simulink model "baseline_super"  (R2021a)
settings: Solver=FixedStepAuto  StartTime=0.0  StopTime=50  FixedStep=framePeriod_s  RelTol=1e-3
undefined symbols (not defined in the file or in its folder): Aircraft, Earth, framePeriod_s, WGS84
libraries: pid_lib x32, simulink x29, aerolibtransform2 x3, simulink_extras x2, aerolibguid x1
(part 2 of 4)

== system baseline_super/RTL CONTROLLER/Horizontal_position_controller ==
  dist_to_tar_m : Inport
  bearing_to_tar_rad : Inport  Port=2
  cur_heading_rad : Inport  Port=3
  Constant : Constant  Value=0  OutDataTypeStr=single
  Constant1 : Constant  Value=Aircraft.Control.v_hor_max  OutDataTypeStr=single
  Constant3 : Constant  Value=0.5  OutDataTypeStr=single
  Mux : Mux  Inputs=2
  PID Controller2 : pid_lib/PID Controller  Controller=P  Form=Parallel  TimeDomain=Discrete-time  UseExternalTs=off  SampleTime=framePeriod_s  IntegratorMethod=Forward Euler  FilterMethod=Forward Euler  ControllerParametersSource=external  P=0.335  I=0.005  D=0  UseFilter=off  N=100  TunerSelectOption=Transfer Function Based (PID Tuner App)  InitialConditionSource=internal  InitialConditionForIntegrator=0  InitialConditionForFilter=0  DifferentiatorICPrevScaledInput=0  ExternalReset=none  TrackingMode=off  Kt=1  LimitOutput=on  SatLimitsSource=external  UpperSaturationLimit=inf  LowerSaturationLimit=-inf  LinearizeAsGain=off  AntiWindupMode=clamping  Kb=1  POutMin=[]  POutMax=[]  IOutMin=[]  IOutMax=[]  DOutMin=[]  DOutMax=[]  NOutMin=[]  NOutMax=[]  SumOutMin=[]  SumOutMax=[]  SaturationOutMin=[]  SaturationOutMax=[]  PParamMin=[]  PParamMax=[]  IParamMin=[]  IParamMax=[]  DParamMin=[]  DParamMax=[]  NParamMin=[]  NParamMax=[]  KbParamMin=[]  KbParamMax=[]  KtParamMin=[]  KtParamMax=[]  KbOutMin=[]  KbOutMax=[]  KtOutMin=[]  KtOutMax=[]  IntegratorOutMin=[]  IntegratorOutMax=[]  FilterOutMin=[]  FilterOutMax=[]  SumI1OutMin=[]  SumI1OutMax=[]  SumI2OutMin=[]  SumI2OutMax=[]  SumI3OutMin=[]  SumI3OutMax=[]  SumI4OutMin=[]  SumI4OutMax=[]  SumDOutMin=[]  SumDOutMax=[]  DifferentiatorOutMin=[]  DifferentiatorOutMax=[]  FilterDiffOutCoefMin=[]  FilterDiffOutCoefMax=[]  ReciprocalOutMin=[]  ReciprocalOutMax=[]  SumDenOutMin=[]  SumDenOutMax=[]  SumNumOutMin=[]  SumNumOutMax=[]  DivideOutMin=[]  DivideOutMax=[]  UdiffTsProdOutMin=[]  UdiffTsProdOutMax=[]  NTsProdOutMin=[]  NTsProdOutMax=[]  UintegralTsProdOutMin=[]  UintegralTsProdOutMax=[]  UngainTsProdOutMin=[]  UngainTsProdOutMax=[]  IntegratorContinuousStateAttributes=''  IntegratorStateMustResolveToSignalObject=off  IntegratorRTWStateStorageClass=Auto  FilterContinuousStateAttributes=''  FilterStateMustResolveToSignalObject=off  FilterRTWStateStorageClass=Auto  ParallelPVariant=ExternalParameters  IdealPVariant=Disabled  IVariant=Disabled  DVariant=Disabled  IntegratorVariant=Disabled  SatVariant=External  AWVariant=Disabled  PCopyVariant=Disabled  TRVariant=Disabled  FdbkBlocksVariant=Forward  IdealPFdbkVariant=Disabled  SatFdbkVariant=Disabled  DerivativeFilterVariant=Disabled  NVariant=Disabled  NCopyVariant=Disabled_SignalSpec  FilterICVariant=Disabled  IntegratorICVariant=Disabled  ExternalResetVariant=Disabled  TRSumVariant=Passthrough  SumFdbkVariant=Disabled  SumVariant=Passthrough_P  TsampFilterVariant=InternalTs  TsampNgainVariant=Passthrough  TsampIntegralVariant=Disabled_SignalSpec  ExternalSaturationOutDataTypeStr=Inherit: Same as second input
  Saturation : Saturate  UpperLimit=20  LowerLimit=0
  convert to ve_cmd : Subsystem
  inertial_to_body conversion : Subsystem
  vb_x : Outport
  vb_y : Outport  Port=2
  wires:
  Constant3/1 -> PID Controller2/2
  cur_heading_rad/1 -> inertial_to_body conversion/2(heading_rad)
  bearing_to_tar_rad/1 -> convert to ve_cmd/2(bearing_to_target_rad)
  convert to ve_cmd/1(ve_x_cmd) -> Mux/1  "ve_x"
  convert to ve_cmd/2(ve_y_cmd) -> Mux/2  "ve_y"
  Mux/1 -> inertial_to_body conversion/1(ve_xy)
  Constant1/1 -> PID Controller2/3
  Constant/1 -> PID Controller2/4
  PID Controller2/1 -> convert to ve_cmd/1(speed_cmd_mps)
  Saturation/1 -> PID Controller2/1
  dist_to_tar_m/1 -> Saturation/1
  inertial_to_body conversion/1(vb_x) -> vb_x/1
  inertial_to_body conversion/2(vb_y) -> vb_y/1

== system baseline_super/RTL CONTROLLER/Trigger Land ==
  Trigger : TriggerPort  VariantControl=(inherit)  PortDimensions=1
  Data Store Write : DataStoreWrite  DataStoreName=cur_mode  IndexOptions=Index vector (dialog)  Indices=1  OutputSizes=1
  Land_mode : Constant  Value=4  OutDataTypeStr=int8
  wires:
  Land_mode/1 -> Data Store Write/1

== system baseline_super/RTL CONTROLLER/heading_controller ==
  Sys_input : Inport
  Bus Selector4 : BusSelector  OutputSignals=Navigation Filter Data.gyro_radps
  Constant : Constant  Value=0  OutDataTypeStr=single
  Selector2 : Selector  InputPortWidth=3  IndexOptions=Index vector (dialog)  Indices=3  OutputSizes=1
  yaw_rate_controller : Subsystem
  yaw_cc : Outport
  wires:
  Bus Selector4/1 -> Selector2/1  "<gyro_radps>"
  Sys_input/1 -> Bus Selector4/1
  Constant/1 -> yaw_rate_controller/1(yaw_rate_cmd_radps)
  yaw_rate_controller/1(yaw_cmd) -> yaw_cc/1
  Selector2/1 -> yaw_rate_controller/2(gyro_z_radps)

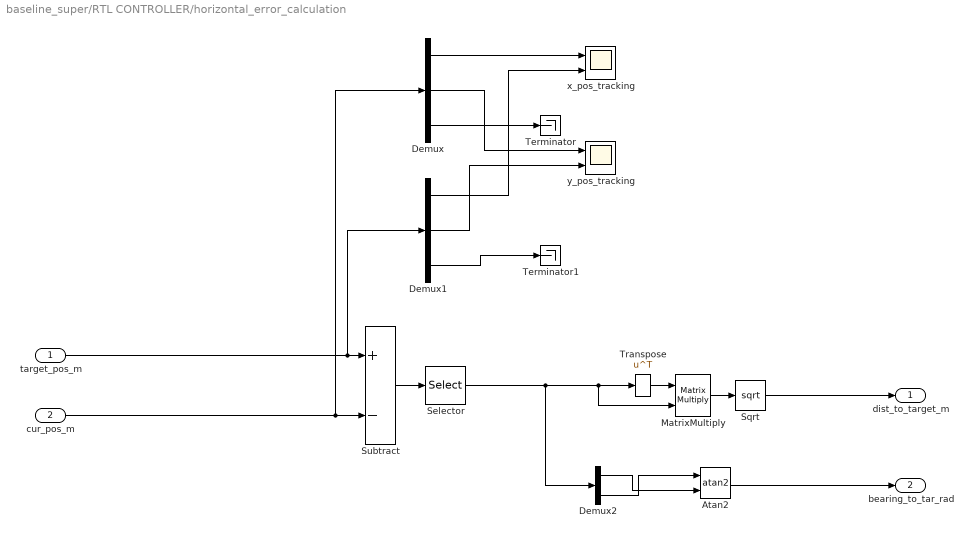
== system baseline_super/RTL CONTROLLER/horizontal_error_calculation  ==
  target_pos_m : Inport
  cur_pos_m : Inport  Port=2
  Atan2 : Trigonometry  Operator=atan2
  Demux : Demux  Outputs=3
  Demux1 : Demux  Outputs=3
  Demux2 : Demux  Outputs=2
  MatrixMultiply : Product  Multiplication=Matrix(*)
  Selector : Selector  InputPortWidth=3  IndexOptions=Index vector (dialog)  Indices=[1 2]  OutputSizes=1
  Sqrt : Sqrt  SaturateOnIntegerOverflow=on
  Subtract : Sum  Inputs=+-
  Terminator : Terminator
  Terminator1 : Terminator
  Transpose : Math  Operator=transpose  SaturateOnIntegerOverflow=on
  x_pos_tracking : Scope  NumInputPorts=2
  y_pos_tracking : Scope  NumInputPorts=2
  dist_to_target_m : Outport
  bearing_to_tar_rad : Outport  Port=2
  wires:
  Demux/3 -> Terminator/1
  Demux/2 -> y_pos_tracking/1
  target_pos_m/1 -> Demux1/1, Subtract/1
  cur_pos_m/1 -> Demux/1, Subtract/2
  Selector/1 -> Demux2/1, MatrixMultiply/2, Transpose/1
  Demux1/3 -> Terminator1/1
  Atan2/1 -> bearing_to_tar_rad/1
  Subtract/1 -> Selector/1
  Demux/1 -> x_pos_tracking/1
  Demux2/2 -> Atan2/1
  Transpose/1 -> MatrixMultiply/1
  Demux1/1 -> x_pos_tracking/2
  Demux1/2 -> y_pos_tracking/2
  MatrixMultiply/1 -> Sqrt/1
  Demux2/1 -> Atan2/2
  Sqrt/1 -> dist_to_target_m/1

== system baseline_super/RTL CONTROLLER/horizontal_speed_controller ==
  vb_x cmd : Inport
  vb_y cmd : Inport  Port=2
  <heading_rad> : Inport  Port=3
  ve_xy : Inport  Port=4
  inertial_to_body conversion : Subsystem
  vb_x_controller : Subsystem
  vb_y_controller : Subsystem
  roll_cmd_rad : Outport
  pitch_cmd_rad : Outport  Port=2
  wires:
  vb_x cmd/1 -> vb_x_controller/1(vb_x cmd)
  vb_y cmd/1 -> vb_y_controller/1(vb_y cmd)
  vb_x_controller/1(pitch_cmd_rad) -> pitch_cmd_rad/1
  vb_y_controller/1(roll_cmd_rad) -> roll_cmd_rad/1
  <heading_rad>/1 -> inertial_to_body conversion/1(<heading_rad>)
  ve_xy/1 -> inertial_to_body conversion/2(ve_xy)
  inertial_to_body conversion/1(vb_y) -> vb_y_controller/2(vb_y)
  inertial_to_body conversion/2(vb_x) -> vb_x_controller/2(vb_x)

== system baseline_super/RTL CONTROLLER/pitch_roll_angle_controller ==
  roll_cmd_rad : Inport
  roll_rad : Inport  Port=2
  pitch_cmd_rad : Inport  Port=3
  pitch_rad : Inport  Port=4
  Pitch Controller : Subsystem
  Roll Controller : Subsystem
  roll_cc : Outport
  pitch_cc : Outport  Port=2
  wires:
  Pitch Controller/1(pitch_cc) -> pitch_cc/1  "pitch_cc"
  pitch_rad/1 -> Pitch Controller/2(pitch_rad)
  Roll Controller/1(roll_cc) -> roll_cc/1  "roll_cc"
  pitch_cmd_rad/1 -> Pitch Controller/1(pitch_cmd_rad)
  roll_cmd_rad/1 -> Roll Controller/1(roll_cmd_rad)
  roll_rad/1 -> Roll Controller/2(roll_rad)

== system baseline_super/RTL CONTROLLER/vertical_position_controller ==
  target_z_m : Inport
  cur_z_m : Inport  Port=2
  Abs : Abs
  Compare To Constant : simulink/Logic and Bit Operations/Compare To Constant  relop=<=  const=Aircraft.Control.wp_radius  OutDataTypeStr=boolean
  Constant : Constant  Value=Aircraft.Control.v_z_up_max  OutDataTypeStr=single
  Constant1 : Constant  Value=Aircraft.Control.v_z_down_max  OutDataTypeStr=single
  Gain : Gain  Gain=-1
  PID Controller2 : pid_lib/PID Controller  Controller=P  Form=Parallel  TimeDomain=Discrete-time  UseExternalTs=off  SampleTime=framePeriod_s  IntegratorMethod=Forward Euler  FilterMethod=Forward Euler  ControllerParametersSource=external  P=0  I=0  D=0  UseFilter=off  N=100  TunerSelectOption=Frequency Response Based  ZeroCross=off  InitialConditionSource=internal  InitialConditionForIntegrator=0  InitialConditionForFilter=0  DifferentiatorICPrevScaledInput=0  ExternalReset=none  TrackingMode=off  Kt=1  LimitOutput=on  SatLimitsSource=external  UpperSaturationLimit=Aircraft.Control.v_z_up_max  LowerSaturationLimit=-Aircraft.Control.v_z_down_max  LinearizeAsGain=on  AntiWindupMode=clamping  Kb=1  POutMin=[]  POutMax=[]  IOutMin=[]  IOutMax=[]  DOutMin=[]  DOutMax=[]  NOutMin=[]  NOutMax=[]  SumOutMin=[]  SumOutMax=[]  SaturationOutMin=[]  SaturationOutMax=[]  PParamMin=[]  PParamMax=[]  IParamMin=[]  IParamMax=[]  DParamMin=[]  DParamMax=[]  NParamMin=[]  NParamMax=[]  KbParamMin=[]  KbParamMax=[]  KtParamMin=[]  KtParamMax=[]  KbOutMin=[]  KbOutMax=[]  KtOutMin=[]  KtOutMax=[]  IntegratorOutMin=[]  IntegratorOutMax=[]  FilterOutMin=[]  FilterOutMax=[]  SumI1OutMin=[]  SumI1OutMax=[]  SumI2OutMin=[]  SumI2OutMax=[]  SumI3OutMin=[]  SumI3OutMax=[]  SumI4OutMin=[]  SumI4OutMax=[]  SumDOutMin=[]  SumDOutMax=[]  DifferentiatorOutMin=[]  DifferentiatorOutMax=[]  FilterDiffOutCoefMin=[]  FilterDiffOutCoefMax=[]  ReciprocalOutMin=[]  ReciprocalOutMax=[]  SumDenOutMin=[]  SumDenOutMax=[]  SumNumOutMin=[]  SumNumOutMax=[]  DivideOutMin=[]  DivideOutMax=[]  UdiffTsProdOutMin=[]  UdiffTsProdOutMax=[]  NTsProdOutMin=[]  NTsProdOutMax=[]  UintegralTsProdOutMin=[]  UintegralTsProdOutMax=[]  UngainTsProdOutMin=[]  UngainTsProdOutMax=[]  IntegratorContinuousStateAttributes=''  IntegratorStateMustResolveToSignalObject=off  IntegratorRTWStateStorageClass=Auto  FilterContinuousStateAttributes=''  FilterStateMustResolveToSignalObject=off  FilterRTWStateStorageClass=Auto  ParallelPVariant=ExternalParameters  IdealPVariant=Disabled  IVariant=Disabled  DVariant=Disabled  IntegratorVariant=Disabled  SatVariant=External  AWVariant=Disabled  PCopyVariant=Disabled  TRVariant=Disabled  FdbkBlocksVariant=Forward  IdealPFdbkVariant=Disabled  SatFdbkVariant=Disabled  DerivativeFilterVariant=Disabled  NVariant=Disabled  NCopyVariant=Disabled_SignalSpec  FilterICVariant=Disabled  IntegratorICVariant=Disabled  ExternalResetVariant=Disabled  TRSumVariant=Passthrough  SumFdbkVariant=Disabled  SumVariant=Passthrough_P  TsampFilterVariant=InternalTs  TsampNgainVariant=Passthrough  TsampIntegralVariant=Disabled_SignalSpec  ExternalSaturationOutDataTypeStr=Inherit: Same as second input
  P_vz1 : Constant  Value=Aircraft.Control.P_alt  OutDataTypeStr=single
  Sum3 : Sum  Inputs=|+-
  ve_z_cmd : Outport
  rtl_alt_cleared : Outport  Port=2
  wires:
  P_vz1/1 -> PID Controller2/2
  target_z_m/1 -> Sum3/1
  Sum3/1 -> Abs/1, PID Controller2/1
  cur_z_m/1 -> Sum3/2
  Constant1/1 -> PID Controller2/3
  Constant/1 -> Gain/1
  Gain/1 -> PID Controller2/4
  PID Controller2/1 -> ve_z_cmd/1
  Compare To Constant/1 -> rtl_alt_cleared/1
  Abs/1 -> Compare To Constant/1

== system baseline_super/RTL CONTROLLER/vertical_speed_controller ==
  ve_z_cmd : Inport
  ve_z_mps : Inport  Port=2
  Constant2 : Constant  Value=Aircraft.Control.est_hover_thr  OutDataTypeStr=single
  D_vz : Constant  Value=Aircraft.Control.D_v_z  OutDataTypeStr=single
  Gain : Gain  Gain=-1
  I_vz : Constant  Value=Aircraft.Control.I_v_z  OutDataTypeStr=single
  PID Controller : pid_lib/PID Controller  Controller=PID  Form=Parallel  TimeDomain=Discrete-time  UseExternalTs=off  SampleTime=framePeriod_s  IntegratorMethod=Forward Euler  FilterMethod=Forward Euler  ControllerParametersSource=external  P=0  I=0  D=0  UseFilter=off  N=100  TunerSelectOption=Frequency Response Based  InitialConditionSource=internal  InitialConditionForIntegrator=0  InitialConditionForFilter=0  DifferentiatorICPrevScaledInput=0  ExternalReset=none  TrackingMode=off  Kt=1  LimitOutput=on  SatLimitsSource=internal  UpperSaturationLimit=inf  LowerSaturationLimit=-inf  LinearizeAsGain=on  AntiWindupMode=clamping  Kb=1  POutMin=[]  POutMax=[]  IOutMin=[]  IOutMax=[]  DOutMin=[]  DOutMax=[]  NOutMin=[]  NOutMax=[]  SumOutMin=[]  SumOutMax=[]  SaturationOutMin=[]  SaturationOutMax=[]  PParamMin=[]  PParamMax=[]  IParamMin=[]  IParamMax=[]  DParamMin=[]  DParamMax=[]  NParamMin=[]  NParamMax=[]  KbParamMin=[]  KbParamMax=[]  KtParamMin=[]  KtParamMax=[]  KbOutMin=[]  KbOutMax=[]  KtOutMin=[]  KtOutMax=[]  IntegratorOutMin=[]  IntegratorOutMax=[]  FilterOutMin=[]  FilterOutMax=[]  SumI1OutMin=[]  SumI1OutMax=[]  SumI2OutMin=[]  SumI2OutMax=[]  SumI3OutMin=[]  SumI3OutMax=[]  SumI4OutMin=[]  SumI4OutMax=[]  SumDOutMin=[]  SumDOutMax=[]  DifferentiatorOutMin=[]  DifferentiatorOutMax=[]  FilterDiffOutCoefMin=[]  FilterDiffOutCoefMax=[]  ReciprocalOutMin=[]  ReciprocalOutMax=[]  SumDenOutMin=[]  SumDenOutMax=[]  SumNumOutMin=[]  SumNumOutMax=[]  DivideOutMin=[]  DivideOutMax=[]  UdiffTsProdOutMin=[]  UdiffTsProdOutMax=[]  NTsProdOutMin=[]  NTsProdOutMax=[]  UintegralTsProdOutMin=[]  UintegralTsProdOutMax=[]  UngainTsProdOutMin=[]  UngainTsProdOutMax=[]  IntegratorContinuousStateAttributes=''  IntegratorStateMustResolveToSignalObject=off  IntegratorRTWStateStorageClass=Auto  FilterContinuousStateAttributes=''  FilterStateMustResolveToSignalObject=off  FilterRTWStateStorageClass=Auto  ParallelPVariant=ExternalParameters  IdealPVariant=Disabled  IVariant=ExternalParameters  DVariant=ExternalParameters  IntegratorVariant=Discrete  SatVariant=Enabled  AWVariant=DiscClampingParallel  PCopyVariant=Disabled  TRVariant=Disabled  FdbkBlocksVariant=Forward  IdealPFdbkVariant=Disabled  SatFdbkVariant=Disabled  DerivativeFilterVariant=Differentiator  NVariant=Passthrough  NCopyVariant=Disabled_SignalSpec  FilterICVariant=InternalICsDifferentiator  IntegratorICVariant=InternalICs  ExternalResetVariant=Disabled  TRSumVariant=Passthrough  SumFdbkVariant=Disabled  SumVariant=Sum_PID  TsampFilterVariant=InternalTs  TsampNgainVariant=Passthrough  TsampIntegralVariant=Passthrough  ExternalSaturationOutDataTypeStr=Inherit: Same as second input
  P_vz : Constant  Value=Aircraft.Control.P_v_z  OutDataTypeStr=single
  Saturation : Saturate  UpperLimit=1  LowerLimit=0
  Sum : Sum  Inputs=|+-
  Sum1 : Sum  Inputs=|++
  throttle : Outport
  wires:
  Sum/1 -> Gain/1  "error"
  Constant2/1 -> Sum1/2
  D_vz/1 -> PID Controller/4
  ve_z_mps/1 -> Sum/2
  I_vz/1 -> PID Controller/3
  Sum1/1 -> Saturation/1
  P_vz/1 -> PID Controller/2
  PID Controller/1 -> Sum1/1
  ve_z_cmd/1 -> Sum/1
  Saturation/1 -> throttle/1  "throttle"
  Gain/1 -> PID Controller/1

== system baseline_super/STABILIZED CONTROLER/Pitch Controller ==
  Pitch Bus : Inport
  Pitch_cmd : Inport  Port=2
  Bus Selector : BusSelector  OutputSignals=Navigation Filter Data.pitch_rad
  Constant : Constant  Value=Aircraft.Control.P_pitch_angle  OutDataTypeStr=single
  Constant1 : Constant  Value=Aircraft.Control.I_pitch_angle  OutDataTypeStr=single
  Constant2 : Constant  Value=Aircraft.Control.D_pitch_angle  OutDataTypeStr=single
  Mux : Mux  Inputs=2
  pitch_norm_to_actual : Gain  Gain=-Aircraft.Control.pitch_angle_lim
  stab_pitch_PID : pid_lib/PID Controller  Controller=PID  Form=Parallel  TimeDomain=Discrete-time  UseExternalTs=off  SampleTime=framePeriod_s  IntegratorMethod=Forward Euler  FilterMethod=Forward Euler  ControllerParametersSource=external  P=0.335  I=0.005  D=0  UseFilter=off  N=100  TunerSelectOption=Transfer Function Based (PID Tuner App)  InitialConditionSource=internal  InitialConditionForIntegrator=0  InitialConditionForFilter=0  DifferentiatorICPrevScaledInput=0  ExternalReset=none  TrackingMode=off  Kt=1  LimitOutput=on  SatLimitsSource=internal  UpperSaturationLimit=inf  LowerSaturationLimit=-inf  LinearizeAsGain=on  AntiWindupMode=clamping  Kb=1  POutMin=[]  POutMax=[]  IOutMin=[]  IOutMax=[]  DOutMin=[]  DOutMax=[]  NOutMin=[]  NOutMax=[]  SumOutMin=[]  SumOutMax=[]  SaturationOutMin=[]  SaturationOutMax=[]  PParamMin=[]  PParamMax=[]  IParamMin=[]  IParamMax=[]  DParamMin=[]  DParamMax=[]  NParamMin=[]  NParamMax=[]  KbParamMin=[]  KbParamMax=[]  KtParamMin=[]  KtParamMax=[]  KbOutMin=[]  KbOutMax=[]  KtOutMin=[]  KtOutMax=[]  IntegratorOutMin=[]  IntegratorOutMax=[]  FilterOutMin=[]  FilterOutMax=[]  SumI1OutMin=[]  SumI1OutMax=[]  SumI2OutMin=[]  SumI2OutMax=[]  SumI3OutMin=[]  SumI3OutMax=[]  SumI4OutMin=[]  SumI4OutMax=[]  SumDOutMin=[]  SumDOutMax=[]  DifferentiatorOutMin=[]  DifferentiatorOutMax=[]  FilterDiffOutCoefMin=[]  FilterDiffOutCoefMax=[]  ReciprocalOutMin=[]  ReciprocalOutMax=[]  SumDenOutMin=[]  SumDenOutMax=[]  SumNumOutMin=[]  SumNumOutMax=[]  DivideOutMin=[]  DivideOutMax=[]  UdiffTsProdOutMin=[]  UdiffTsProdOutMax=[]  NTsProdOutMin=[]  NTsProdOutMax=[]  UintegralTsProdOutMin=[]  UintegralTsProdOutMax=[]  UngainTsProdOutMin=[]  UngainTsProdOutMax=[]  IntegratorContinuousStateAttributes=''  IntegratorStateMustResolveToSignalObject=off  IntegratorRTWStateStorageClass=Auto  FilterContinuousStateAttributes=''  FilterStateMustResolveToSignalObject=off  FilterRTWStateStorageClass=Auto  ParallelPVariant=ExternalParameters  IdealPVariant=Disabled  IVariant=ExternalParameters  DVariant=ExternalParameters  IntegratorVariant=Discrete  SatVariant=Enabled  AWVariant=DiscClampingParallel  PCopyVariant=Disabled  TRVariant=Disabled  FdbkBlocksVariant=Forward  IdealPFdbkVariant=Disabled  SatFdbkVariant=Disabled  DerivativeFilterVariant=Differentiator  NVariant=Passthrough  NCopyVariant=Disabled_SignalSpec  FilterICVariant=InternalICsDifferentiator  IntegratorICVariant=InternalICs  ExternalResetVariant=Disabled  TRSumVariant=Passthrough  SumFdbkVariant=Disabled  SumVariant=Sum_PID  TsampFilterVariant=InternalTs  TsampNgainVariant=Passthrough  TsampIntegralVariant=Passthrough  ExternalSaturationOutDataTypeStr=Inherit: Same as second input
  stab_pitch_angle_error_calc : Sum  Inputs=|+-
  stab_pitch_rate_saturation : Saturate  UpperLimit=Aircraft.Control.pitch_rate_max  LowerLimit=-Aircraft.Control.pitch_rate_max  LinearizeAsGain=off
  pitch_cc : Outport
  Logging : Outport  Port=2
  wires:
  stab_pitch_angle_error_calc/1 -> stab_pitch_PID/1  "pitch error"
  Pitch Bus/1 -> Bus Selector/1
  Bus Selector/1 -> Mux/2, stab_pitch_angle_error_calc/2  "<pitch_rad>"
  pitch_norm_to_actual/1 -> Mux/1, stab_pitch_angle_error_calc/1  "pitch angle cmd"
  stab_pitch_PID/1 -> stab_pitch_rate_saturation/1
  Constant2/1 -> stab_pitch_PID/4  "D_gain"
  Constant1/1 -> stab_pitch_PID/3  "I_gain"
  Constant/1 -> stab_pitch_PID/2  "P_gain"
  Pitch_cmd/1 -> pitch_norm_to_actual/1
  Mux/1 -> Logging/1
  stab_pitch_rate_saturation/1 -> pitch_cc/1

== system baseline_super/STABILIZED CONTROLER/Roll Controller ==
  Roll Bus : Inport
  Roll_cmd : Inport  Port=2
  Bus Selector : BusSelector  OutputSignals=Navigation Filter Data.roll_rad
  Constant : Constant  Value=Aircraft.Control.P_roll_angle  OutDataTypeStr=single
  Constant1 : Constant  Value=Aircraft.Control.I_roll_angle  OutDataTypeStr=single
  Constant2 : Constant  Value=Aircraft.Control.D_roll_angle  OutDataTypeStr=single
  Mux : Mux  Inputs=2
  roll_norm_to_actual : Gain  Gain=Aircraft.Control.roll_angle_lim
  stab_roll_PID : pid_lib/PID Controller  Controller=PID  Form=Parallel  TimeDomain=Discrete-time  UseExternalTs=off  SampleTime=framePeriod_s  IntegratorMethod=Forward Euler  FilterMethod=Forward Euler  ControllerParametersSource=external  P=0.335  I=0.005  D=0  UseFilter=off  N=100  TunerSelectOption=Transfer Function Based (PID Tuner App)  InitialConditionSource=internal  InitialConditionForIntegrator=0  InitialConditionForFilter=0  DifferentiatorICPrevScaledInput=0  ExternalReset=none  TrackingMode=off  Kt=1  LimitOutput=on  SatLimitsSource=internal  UpperSaturationLimit=inf  LowerSaturationLimit=-inf  LinearizeAsGain=on  AntiWindupMode=clamping  Kb=1  POutMin=[]  POutMax=[]  IOutMin=[]  IOutMax=[]  DOutMin=[]  DOutMax=[]  NOutMin=[]  NOutMax=[]  SumOutMin=[]  SumOutMax=[]  SaturationOutMin=[]  SaturationOutMax=[]  PParamMin=[]  PParamMax=[]  IParamMin=[]  IParamMax=[]  DParamMin=[]  DParamMax=[]  NParamMin=[]  NParamMax=[]  KbParamMin=[]  KbParamMax=[]  KtParamMin=[]  KtParamMax=[]  KbOutMin=[]  KbOutMax=[]  KtOutMin=[]  KtOutMax=[]  IntegratorOutMin=[]  IntegratorOutMax=[]  FilterOutMin=[]  FilterOutMax=[]  SumI1OutMin=[]  SumI1OutMax=[]  SumI2OutMin=[]  SumI2OutMax=[]  SumI3OutMin=[]  SumI3OutMax=[]  SumI4OutMin=[]  SumI4OutMax=[]  SumDOutMin=[]  SumDOutMax=[]  DifferentiatorOutMin=[]  DifferentiatorOutMax=[]  FilterDiffOutCoefMin=[]  FilterDiffOutCoefMax=[]  ReciprocalOutMin=[]  ReciprocalOutMax=[]  SumDenOutMin=[]  SumDenOutMax=[]  SumNumOutMin=[]  SumNumOutMax=[]  DivideOutMin=[]  DivideOutMax=[]  UdiffTsProdOutMin=[]  UdiffTsProdOutMax=[]  NTsProdOutMin=[]  NTsProdOutMax=[]  UintegralTsProdOutMin=[]  UintegralTsProdOutMax=[]  UngainTsProdOutMin=[]  UngainTsProdOutMax=[]  IntegratorContinuousStateAttributes=''  IntegratorStateMustResolveToSignalObject=off  IntegratorRTWStateStorageClass=Auto  FilterContinuousStateAttributes=''  FilterStateMustResolveToSignalObject=off  FilterRTWStateStorageClass=Auto  ParallelPVariant=ExternalParameters  IdealPVariant=Disabled  IVariant=ExternalParameters  DVariant=ExternalParameters  IntegratorVariant=Discrete  SatVariant=Enabled  AWVariant=DiscClampingParallel  PCopyVariant=Disabled  TRVariant=Disabled  FdbkBlocksVariant=Forward  IdealPFdbkVariant=Disabled  SatFdbkVariant=Disabled  DerivativeFilterVariant=Differentiator  NVariant=Passthrough  NCopyVariant=Disabled_SignalSpec  FilterICVariant=InternalICsDifferentiator  IntegratorICVariant=InternalICs  ExternalResetVariant=Disabled  TRSumVariant=Passthrough  SumFdbkVariant=Disabled  SumVariant=Sum_PID  TsampFilterVariant=InternalTs  TsampNgainVariant=Passthrough  TsampIntegralVariant=Passthrough  ExternalSaturationOutDataTypeStr=Inherit: Same as second input
  stab_roll_angle_error_calc : Sum  Inputs=|+-
  stab_roll_rate_saturation : Saturate  UpperLimit=Aircraft.Control.roll_rate_max  LowerLimit=-Aircraft.Control.roll_rate_max
  roll_cc : Outport
  Logging : Outport  Port=2
  wires:
  stab_roll_PID/1 -> stab_roll_rate_saturation/1  "Roll_cmd"
  roll_norm_to_actual/1 -> Mux/1, stab_roll_angle_error_calc/1  "roll_angle_command"
  stab_roll_angle_error_calc/1 -> stab_roll_PID/1  "roll_angle_error"
  Roll Bus/1 -> Bus Selector/1
  Bus Selector/1 -> Mux/2, stab_roll_angle_error_calc/2  "<roll_rad>"
  Constant/1 -> stab_roll_PID/2  "P_gain"
  Constant1/1 -> stab_roll_PID/3  "I_gain"
  Constant2/1 -> stab_roll_PID/4  "D_gain"
  Roll_cmd/1 -> roll_norm_to_actual/1
  Mux/1 -> Logging/1
  stab_roll_rate_saturation/1 -> roll_cc/1

== system baseline_super/STABILIZED CONTROLER/Yaw Rate Controller ==
  Yaw Bus : Inport
  Yaw_cmd : Inport  Port=2
  Bus Selector : BusSelector  OutputSignals=Navigation Filter Data.gyro_radps
  Constant : Constant  Value=Aircraft.Control.P_yaw_rate  OutDataTypeStr=single
  Constant1 : Constant  Value=Aircraft.Control.I_yaw_rate  OutDataTypeStr=single
  Constant2 : Constant  Value=Aircraft.Control.D_yaw_rate  OutDataTypeStr=single
  Mux : Mux  Inputs=2
  Selector : Selector  InputPortWidth=3  IndexOptions=Index vector (dialog)  Indices=3  OutputSizes=1
  stab_yaw_rate_PID : pid_lib/PID Controller  Controller=PID  Form=Parallel  TimeDomain=Discrete-time  UseExternalTs=off  SampleTime=framePeriod_s  IntegratorMethod=Forward Euler  FilterMethod=Forward Euler  ControllerParametersSource=external  P=1.85  I=0.01  D=0  UseFilter=off  N=100  TunerSelectOption=Transfer Function Based (PID Tuner App)  InitialConditionSource=internal  InitialConditionForIntegrator=0  InitialConditionForFilter=0  DifferentiatorICPrevScaledInput=0  ExternalReset=none  TrackingMode=off  Kt=1  LimitOutput=on  SatLimitsSource=internal  UpperSaturationLimit=inf  LowerSaturationLimit=-inf  LinearizeAsGain=off  AntiWindupMode=clamping  Kb=1  POutMin=[]  POutMax=[]  IOutMin=[]  IOutMax=[]  DOutMin=[]  DOutMax=[]  NOutMin=[]  NOutMax=[]  SumOutMin=[]  SumOutMax=[]  SaturationOutMin=[]  SaturationOutMax=[]  PParamMin=[]  PParamMax=[]  IParamMin=[]  IParamMax=[]  DParamMin=[]  DParamMax=[]  NParamMin=[]  NParamMax=[]  KbParamMin=[]  KbParamMax=[]  KtParamMin=[]  KtParamMax=[]  KbOutMin=[]  KbOutMax=[]  KtOutMin=[]  KtOutMax=[]  IntegratorOutMin=[]  IntegratorOutMax=[]  FilterOutMin=[]  FilterOutMax=[]  SumI1OutMin=[]  SumI1OutMax=[]  SumI2OutMin=[]  SumI2OutMax=[]  SumI3OutMin=[]  SumI3OutMax=[]  SumI4OutMin=[]  SumI4OutMax=[]  SumDOutMin=[]  SumDOutMax=[]  DifferentiatorOutMin=[]  DifferentiatorOutMax=[]  FilterDiffOutCoefMin=[]  FilterDiffOutCoefMax=[]  ReciprocalOutMin=[]  ReciprocalOutMax=[]  SumDenOutMin=[]  SumDenOutMax=[]  SumNumOutMin=[]  SumNumOutMax=[]  DivideOutMin=[]  DivideOutMax=[]  UdiffTsProdOutMin=[]  UdiffTsProdOutMax=[]  NTsProdOutMin=[]  NTsProdOutMax=[]  UintegralTsProdOutMin=[]  UintegralTsProdOutMax=[]  UngainTsProdOutMin=[]  UngainTsProdOutMax=[]  IntegratorContinuousStateAttributes=''  IntegratorStateMustResolveToSignalObject=off  IntegratorRTWStateStorageClass=Auto  FilterContinuousStateAttributes=''  FilterStateMustResolveToSignalObject=off  FilterRTWStateStorageClass=Auto  ParallelPVariant=ExternalParameters  IdealPVariant=Disabled  IVariant=ExternalParameters  DVariant=ExternalParameters  IntegratorVariant=Discrete  SatVariant=Enabled  AWVariant=DiscClampingParallel  PCopyVariant=Disabled  TRVariant=Disabled  FdbkBlocksVariant=Forward  IdealPFdbkVariant=Disabled  SatFdbkVariant=Disabled  DerivativeFilterVariant=Differentiator  NVariant=Passthrough  NCopyVariant=Disabled_SignalSpec  FilterICVariant=InternalICsDifferentiator  IntegratorICVariant=InternalICs  ExternalResetVariant=Disabled  TRSumVariant=Passthrough  SumFdbkVariant=Disabled  SumVariant=Sum_PID  TsampFilterVariant=InternalTs  TsampNgainVariant=Passthrough  TsampIntegralVariant=Passthrough  ExternalSaturationOutDataTypeStr=Inherit: Same as second input
  stab_yaw_rate_error_calc : Sum  Inputs=|+-
  yaw_norm_tp_actual : Gain  Gain=Aircraft.Control.yaw_rate_max
  yaw_cc : Outport
  Logging : Outport  Port=2
  wires:
  Yaw Bus/1 -> Bus Selector/1
  yaw_norm_tp_actual/1 -> Mux/1, stab_yaw_rate_error_calc/1
  Selector/1 -> Mux/2, stab_yaw_rate_error_calc/2
  Bus Selector/1 -> Selector/1  "<gyro_radps>"
  stab_yaw_rate_error_calc/1 -> stab_yaw_rate_PID/1
  stab_yaw_rate_PID/1 -> yaw_cc/1
  Constant/1 -> stab_yaw_rate_PID/2
  Constant1/1 -> stab_yaw_rate_PID/3
  Constant2/1 -> stab_yaw_rate_PID/4
  Yaw_cmd/1 -> yaw_norm_tp_actual/1
  Mux/1 -> Logging/1

== system baseline_super/To VMS Data/SBUS & AUX1 ==
  Bus Creator : BusCreator  Inputs=4  OutDataTypeStr=Bus: SbusCmd  NonVirtualBus=on
  Cast To Boolean : DataTypeConversion  OutDataTypeStr=boolean
  Cast To Boolean1 : DataTypeConversion  OutDataTypeStr=boolean
  Cast To Single : DataTypeConversion  OutDataTypeStr=single
  Cast To Single1 : DataTypeConversion  OutDataTypeStr=int16
  Constant : Constant  Value=0  OutDataTypeStr=boolean
  Constant1 : Constant  Value=0  OutDataTypeStr=boolean
  Ground1 : Ground
  Ground2 : Ground
  sbus : Outport  SampleTime=framePeriod_s
  wires:
  Bus Creator/1 -> sbus/1
  Constant/1 -> Cast To Boolean/1  "ch17"
  Constant1/1 -> Cast To Boolean1/1  "ch18"
  Ground2/1 -> Cast To Single/1  "cmd"
  Cast To Boolean/1 -> Bus Creator/1  "ch17"
  Cast To Boolean1/1 -> Bus Creator/2  "ch18"
  Cast To Single/1 -> Bus Creator/4  "cmd"
  Cast To Single1/1 -> Bus Creator/3  "cnt"
  Ground1/1 -> Cast To Single1/1  "cnt"

== system baseline_super/To VMS Data/Subsystem ==
  note: cmd - output to feed to the simulator
  note: cnt - pwm output to actual hardware
  norm_pwm : Inport
  Bus Creator : BusCreator  Inputs=2  OutDataTypeStr=Bus: PwmCmd  NonVirtualBus=on
      settings: InheritFromInputs=off
  Constant : Constant  Value=1000
  Data Type Conversion : DataTypeConversion  OutDataTypeStr=int16
  Gain : Gain  Gain=1000
  Sum : Sum  Inputs=|++
  PwmCmd : Outport
  wires:
  Constant/1 -> Sum/2
  Bus Creator/1 -> PwmCmd/1
  norm_pwm/1 -> Gain/1, Bus Creator/2  "cmd"
  Gain/1 -> Sum/1
  Sum/1 -> Data Type Conversion/1
  Data Type Conversion/1 -> Bus Creator/1  "cnt"

== system baseline_super/WAYPOINT CONTROLLER/WP_NAV ==
  Sys_input : Inport
  Enable : EnablePort
  Bus Creator4 : BusCreator  Inputs=4
  Horizontal position controller : Subsystem
  Vertical position controller : Subsystem
  heading_controller : Subsystem
  Command out : Outport
  wires:
  Bus Creator4/1 -> Command out/1
  Sys_input/1 -> Vertical position controller/1(Sys_input), heading_controller/1(Sys_input), Horizontal position controller/1(Sys_input)
  Vertical position controller/1(throttle_out) -> Bus Creator4/1
  heading_controller/1(yaw_cc) -> Bus Creator4/4  "yaw_cc"
  Horizontal position controller/1(roll_cc) -> Bus Creator4/2  "roll_cc"
  Horizontal position controller/2(pitch_cc) -> Bus Creator4/3  "pitch_cc"

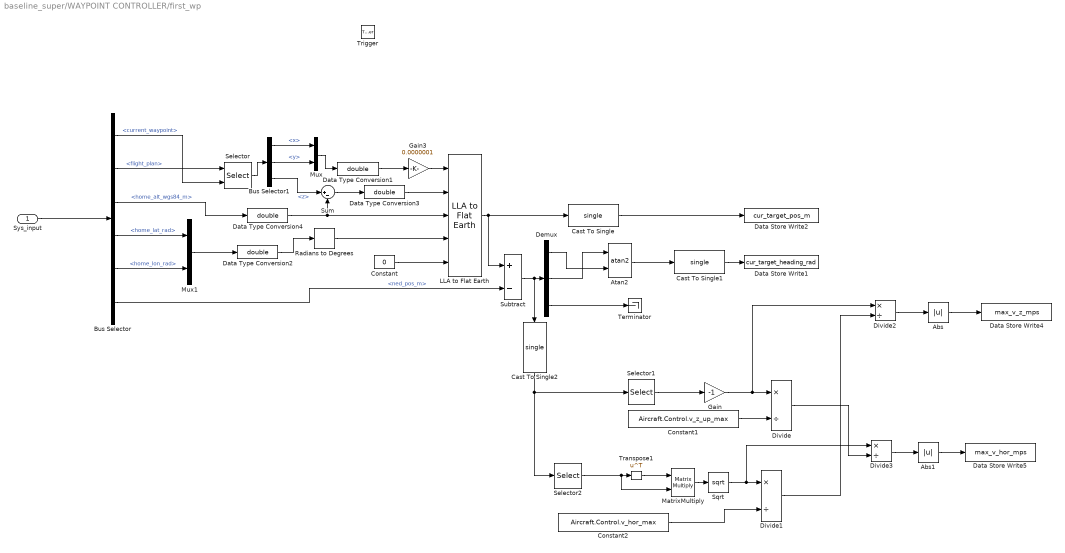
== system baseline_super/WAYPOINT CONTROLLER/first_wp ==
  Sys_input : Inport
  Trigger : TriggerPort  VariantControl=(inherit)  OutputDataType=double  PortDimensions=1
  Abs : Abs
  Abs1 : Abs
  Atan2 : Trigonometry  Operator=atan2
  Bus Selector : BusSelector  OutputSignals=Telemetry Data.current_waypoint,Telemetry Data.flight_plan,Navigation Filter Data.home_alt_wgs84_m,Navigation Filter Data.home_lat_rad,Navigation Filter Data.home_lon_rad,Navigation Filter Data.ned_pos_m
  Bus Selector1 : BusSelector  OutputSignals=x,y,z
  Cast To Single : DataTypeConversion  OutDataTypeStr=single
  Cast To Single1 : DataTypeConversion  OutDataTypeStr=single
  Cast To Single2 : DataTypeConversion  OutDataTypeStr=single
  Constant : Constant  Value=0  OutDataTypeStr=double
  Constant1 : Constant  Value=Aircraft.Control.v_z_up_max  OutDataTypeStr=single
  Constant2 : Constant  Value=Aircraft.Control.v_hor_max  OutDataTypeStr=single
  Data Store Write1 : DataStoreWrite  DataStoreName=cur_target_heading_rad  IndexOptions=Index vector (dialog)  Indices=1  OutputSizes=1
  Data Store Write2 : DataStoreWrite  DataStoreName=cur_target_pos_m  IndexOptions=Index vector (dialog)  Indices=1  OutputSizes=1
  Data Store Write4 : DataStoreWrite  DataStoreName=max_v_z_mps  IndexOptions=Index vector (dialog)  Indices=1  OutputSizes=1
  Data Store Write5 : DataStoreWrite  DataStoreName=max_v_hor_mps  IndexOptions=Index vector (dialog)  Indices=1  OutputSizes=1
  Data Type Conversion{1..4} (4 alike) : DataTypeConversion  OutDataTypeStr=double
  Demux : Demux  Outputs=3
  Divide{,1..3} (4 alike) : Product  Inputs=*/
  Gain : Gain  Gain=-1
  Gain3 : Gain  Gain=0.0000001
  LLA to Flat Earth : aerolibtransform2/LLA to Flat Earth  units=Metric (MKS)  ptype=Earth (WGS84)  F=1/298.257223563  R=6378137  refPosPort=on  LL0=[0 10]  psi=0
      settings: SourceProductBaseCode=AE
  MatrixMultiply : Product  Multiplication=Matrix(*)
  Mux : Mux  Inputs=2
  Mux1 : Mux  Inputs=2
  Radians to Degrees : simulink_extras/Transformations/Radians to Degrees
  Selector : Selector  IndexMode=Zero-based  InputPortWidth=500  IndexOptions=Index vector (port)  Indices=[1 3]  OutputSizes=1
  Selector1 : Selector  InputPortWidth=3  IndexOptions=Index vector (dialog)  Indices=3  OutputSizes=1
  Selector2 : Selector  InputPortWidth=3  IndexOptions=Index vector (dialog)  Indices=[1 2]  OutputSizes=1
  Sqrt : Sqrt  SaturateOnIntegerOverflow=on
  Subtract : Sum  Inputs=+-
  Sum : Sum  Inputs=|+-
  Terminator : Terminator
  Transpose1 : Math  Operator=transpose  SaturateOnIntegerOverflow=on
  wires:
  Bus Selector/1 -> Selector/2  "<current_waypoint>"
  Sys_input/1 -> Bus Selector/1
  Bus Selector/2 -> Selector/1  "<flight_plan>"
  Selector/1 -> Bus Selector1/1
  Bus Selector1/1 -> Mux/1  "<x>"
  Data Type Conversion1/1 -> Gain3/1
  Gain3/1 -> LLA to Flat Earth/1
  Bus Selector1/2 -> Mux/2  "<y>"
  Mux/1 -> Data Type Conversion1/1
  Bus Selector/3 -> Data Type Conversion4/1  "<home_alt_wgs84_m>"
  Constant/1 -> LLA to Flat Earth/5
  Bus Selector/4 -> Mux1/1  "<home_lat_rad>"
  Bus Selector/5 -> Mux1/2  "<home_lon_rad>"
  Mux1/1 -> Data Type Conversion2/1
  Radians to Degrees/1 -> LLA to Flat Earth/4
  LLA to Flat Earth/1 -> Subtract/1, Cast To Single/1
  Bus Selector/6 -> Subtract/2  "<ned_pos_m>"
  Subtract/1 -> Cast To Single2/1, Demux/1
  Demux/3 -> Terminator/1
  Demux/2 -> Atan2/1
  Demux/1 -> Atan2/2
  Atan2/1 -> Cast To Single1/1
  Data Type Conversion2/1 -> Radians to Degrees/1
  Data Type Conversion3/1 -> LLA to Flat Earth/2
  Data Type Conversion4/1 -> Sum/2, LLA to Flat Earth/3
  Bus Selector1/3 -> Sum/1  "<z>"
  Sum/1 -> Data Type Conversion3/1
  Cast To Single/1 -> Data Store Write2/1
  Cast To Single1/1 -> Data Store Write1/1
  Selector1/1 -> Gain/1
  Gain/1 -> Divide/1, Divide2/1
  Constant1/1 -> Divide/2
  Divide/1 -> Divide3/2
  MatrixMultiply/1 -> Sqrt/1
  Constant2/1 -> Divide1/2
  Sqrt/1 -> Divide3/1, Divide1/1
  Divide1/1 -> Divide2/2
  Cast To Single2/1 -> Selector1/1, Selector2/1
  Selector2/1 -> MatrixMultiply/2, Transpose1/1
  Transpose1/1 -> MatrixMultiply/1
  Divide2/1 -> Abs/1
  Divide3/1 -> Abs1/1
  Abs/1 -> Data Store Write4/1
  Abs1/1 -> Data Store Write5/1

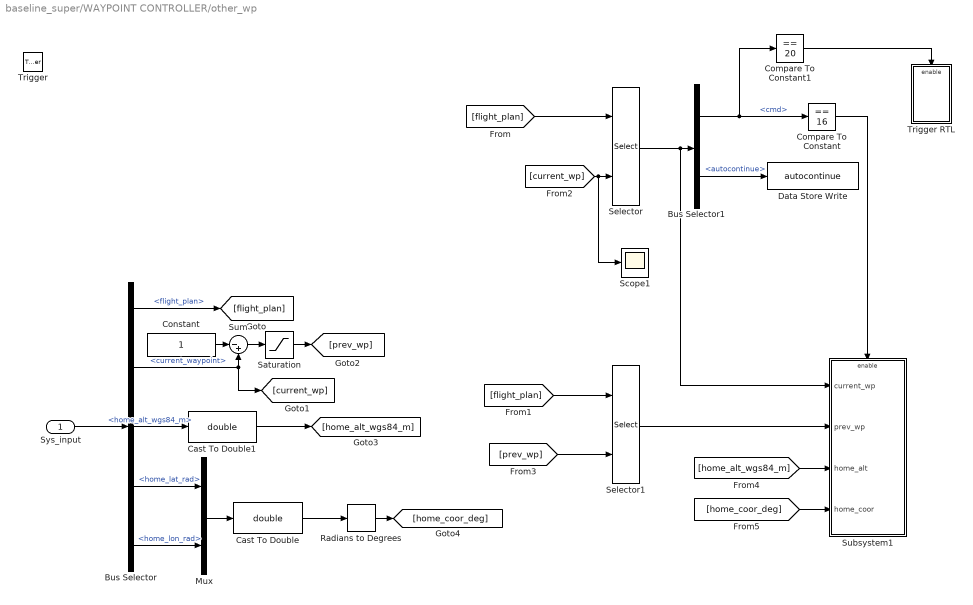
== system baseline_super/WAYPOINT CONTROLLER/other_wp ==
  Sys_input : Inport
  Trigger : TriggerPort  VariantControl=(inherit)  OutputDataType=double  PortDimensions=1
  Bus Selector : BusSelector  OutputSignals=Telemetry Data.flight_plan,Telemetry Data.current_waypoint,Navigation Filter Data.home_alt_wgs84_m,Navigation Filter Data.home_lat_rad,Navigation Filter Data.home_lon_rad
  Bus Selector1 : BusSelector  OutputSignals=cmd,autocontinue
  Cast To Double : DataTypeConversion  OutDataTypeStr=double
  Cast To Double1 : DataTypeConversion  OutDataTypeStr=double
  Compare To Constant : simulink/Logic and Bit Operations/Compare To Constant  relop===  const=16  OutDataTypeStr=boolean
  Compare To Constant1 : simulink/Logic and Bit Operations/Compare To Constant  relop===  const=20  OutDataTypeStr=boolean
  Constant : Constant
  Data Store Write : DataStoreWrite  DataStoreName=autocontinue  IndexOptions=Index vector (dialog)  Indices=1  OutputSizes=1
  Mux : Mux  Inputs=2
  Radians to Degrees : simulink_extras/Transformations/Radians to Degrees
  Saturation : Saturate  UpperLimit=500  LowerLimit=0
  Scope1 : Scope
  Selector : Selector  IndexMode=Zero-based  InputPortWidth=500  IndexOptions=Index vector (port)  Indices=[1 3]  OutputSizes=1
  Selector1 : Selector  IndexMode=Zero-based  InputPortWidth=500  IndexOptions=Index vector (port)  Indices=[1 3]  OutputSizes=1
  Subsystem1 : Subsystem
  Sum : Sum  Inputs=|-+
  Trigger RTL : Subsystem
  wires:
  Sys_input/1 -> Bus Selector/1
  Bus Selector/1 -> [flight_plan]  "<flight_plan>"
  Bus Selector/2 -> Sum/2, [current_wp]  "<current_waypoint>"
  Constant/1 -> Sum/1
  Sum/1 -> Saturation/1
  Saturation/1 -> [prev_wp]
  [flight_plan] -> Selector/1
  [flight_plan] -> Selector1/1
  [current_wp] -> Scope1/1, Selector/2
  Bus Selector/3 -> Cast To Double1/1  "<home_alt_wgs84_m>"
  Bus Selector/4 -> Mux/1  "<home_lat_rad>"
  Bus Selector/5 -> Mux/2  "<home_lon_rad>"
  Radians to Degrees/1 -> [home_coor_deg]
  [prev_wp] -> Selector1/2
  Selector/1 -> Subsystem1/1(current_wp), Bus Selector1/1
  Bus Selector1/1 -> Compare To Constant/1, Compare To Constant1/1  "<cmd>"
  Compare To Constant/1 -> Subsystem1/Enable
  Compare To Constant1/1 -> Trigger RTL/Enable
  Selector1/1 -> Subsystem1/2(prev_wp)
  [home_alt_wgs84_m] -> Subsystem1/3(home_alt)
  [home_coor_deg] -> Subsystem1/4(home_coor)
  Mux/1 -> Cast To Double/1
  Cast To Double/1 -> Radians to Degrees/1
  Cast To Double1/1 -> [home_alt_wgs84_m]
  Bus Selector1/2 -> Data Store Write/1  "<autocontinue>"

== system baseline_super/WAYPOINT CONTROLLER/wp_completion_check ==
  note: Output wp_reached cmd only when distance between current pos and target pos is less than wp_radius and autocontinue is true. Set the mode to Pos_hold if wp_completed and autocontinue is false
  Sys_input : Inport
  AND : Logic  IconShape=distinctive  AllPortsSameDT=off  OutDataTypeStr=boolean
  AND1 : Logic  Inputs=3  IconShape=distinctive  AllPortsSameDT=off  OutDataTypeStr=boolean
  Bus Selector : BusSelector  OutputSignals=Navigation Filter Data.ned_pos_m
  Calculate Range : aerolibguid/Calculate Range
      settings: SourceProductBaseCode=AE
  Compare To Constant : simulink/Logic and Bit Operations/Compare To Constant  relop=<=  const=Aircraft.Control.wp_radius  OutDataTypeStr=boolean
  Compare To Constant1 : simulink/Logic and Bit Operations/Compare To Constant  relop===  const=3  OutDataTypeStr=boolean
  Data Store Read : DataStoreRead  DataStoreName=cur_target_pos_m  IndexOptions=Index vector (dialog)  Indices=1  OutputSizes=1
  Data Store Read1 : DataStoreRead  DataStoreName=autocontinue  IndexOptions=Index vector (dialog)  Indices=1  OutputSizes=1
  Data Store Read2 : DataStoreRead  DataStoreName=cur_mode  IndexOptions=Index vector (dialog)  Indices=1  OutputSizes=1
  NOT : Logic  Operator=NOT  IconShape=distinctive  AllPortsSameDT=off  OutDataTypeStr=boolean
  NOT1 : Logic  Operator=NOT  IconShape=distinctive  AllPortsSameDT=off  OutDataTypeStr=boolean
  Trigger Pos_hold : Subsystem
  wp_reached : Outport
  wires:
  Sys_input/1 -> Bus Selector/1
  Compare To Constant/1 -> AND1/1, AND/1
  Data Store Read1/1 -> NOT/1, AND/2
  NOT/1 -> AND1/2
  AND/1 -> wp_reached/1
  AND1/1 -> Trigger Pos_hold/Trigger
  Data Store Read2/1 -> Compare To Constant1/1
  NOT1/1 -> AND1/3
  Compare To Constant1/1 -> NOT1/1
  Calculate Range/1 -> Compare To Constant/1
  Data Store Read/1 -> Calculate Range/1
  Bus Selector/1 -> Calculate Range/2  "<ned_pos_m>"

== system baseline_super/Failsafe_management/Battery failsafe/Trigger Land ==
  Enable : EnablePort
  Data Store Write : DataStoreWrite  DataStoreName=cur_mode  IndexOptions=Index vector (dialog)  Indices=1  OutputSizes=1
  land_mode : Constant  Value=5  OutDataTypeStr=int8
  wires:
  land_mode/1 -> Data Store Write/1

== system baseline_super/Failsafe_management/Battery failsafe/disarm motor ==
  Enable : EnablePort  StatesWhenEnabling=reset
  Compare To Constant2 : simulink/Logic and Bit Operations/Compare To Constant  relop=>  const=15  OutDataTypeStr=boolean
  Constant : Constant  Value=framePeriod_s
  Sum : Sum  Inputs=|++
  Unit Delay : UnitDelay  SampleTime=-1  HasFrameUpgradeWarning=on
  battery_low_trigger : Outport
  wires:
  Compare To Constant2/1 -> battery_low_trigger/1
  Sum/1 -> Compare To Constant2/1, Unit Delay/1
  Unit Delay/1 -> Sum/2
  Constant/1 -> Sum/1

== system baseline_super/Failsafe_management/Radio failsafe/Trigger RTL ==
  Enable : EnablePort
  Data Store Write : DataStoreWrite  DataStoreName=cur_mode  IndexOptions=Index vector (dialog)  Indices=1  OutputSizes=1
  rtl_mode : Constant  Value=3  OutDataTypeStr=int8
  wires:
  rtl_mode/1 -> Data Store Write/1

== system baseline_super/LAND CONTROLLER/Horizontal speed controller/2D rotation from NED_xy to body_xy ==
  <heading_rad> : Inport
  Cos : Trigonometry  Operator=cos
  Gain : Gain  Gain=-1
  Mux : Mux
  Reshape : Reshape  OutputDimensionality=Customize  OutputDimensions=[2,2]
  Sin : Trigonometry
  2D_rot : Outport
  wires:
  <heading_rad>/1 -> Sin/1, Cos/1
  Mux/1 -> Reshape/1
  Sin/1 -> Mux/3, Gain/1
  Cos/1 -> Mux/1, Mux/4
  Reshape/1 -> 2D_rot/1
  Gain/1 -> Mux/2

== system baseline_super/LAND CONTROLLER/Horizontal speed controller/Pitch Controller ==
  pitch_cmd_rad : Inport
  pitch_rad : Inport  Port=2
  D_pitch_angle : Constant  Value=Aircraft.Control.I_pitch_angle  OutDataTypeStr=single
  I_pitch_angle : Constant  Value=Aircraft.Control.D_pitch_angle  OutDataTypeStr=single
  P_pitch_angle : Constant  Value=Aircraft.Control.P_pitch_angle  OutDataTypeStr=single
  Pitch angle controller : pid_lib/PID Controller  Controller=PID  Form=Parallel  TimeDomain=Discrete-time  UseExternalTs=off  SampleTime=framePeriod_s  IntegratorMethod=Forward Euler  FilterMethod=Forward Euler  ControllerParametersSource=external  P=0.335  I=0.005  D=0  UseFilter=off  N=100  TunerSelectOption=Transfer Function Based (PID Tuner App)  InitialConditionSource=internal  InitialConditionForIntegrator=0  InitialConditionForFilter=0  DifferentiatorICPrevScaledInput=0  ExternalReset=none  TrackingMode=off  Kt=1  LimitOutput=on  SatLimitsSource=internal  UpperSaturationLimit=inf  LowerSaturationLimit=-inf  LinearizeAsGain=off  AntiWindupMode=clamping  Kb=1  POutMin=[]  POutMax=[]  IOutMin=[]  IOutMax=[]  DOutMin=[]  DOutMax=[]  NOutMin=[]  NOutMax=[]  SumOutMin=[]  SumOutMax=[]  SaturationOutMin=[]  SaturationOutMax=[]  PParamMin=[]  PParamMax=[]  IParamMin=[]  IParamMax=[]  DParamMin=[]  DParamMax=[]  NParamMin=[]  NParamMax=[]  KbParamMin=[]  KbParamMax=[]  KtParamMin=[]  KtParamMax=[]  KbOutMin=[]  KbOutMax=[]  KtOutMin=[]  KtOutMax=[]  IntegratorOutMin=[]  IntegratorOutMax=[]  FilterOutMin=[]  FilterOutMax=[]  SumI1OutMin=[]  SumI1OutMax=[]  SumI2OutMin=[]  SumI2OutMax=[]  SumI3OutMin=[]  SumI3OutMax=[]  SumI4OutMin=[]  SumI4OutMax=[]  SumDOutMin=[]  SumDOutMax=[]  DifferentiatorOutMin=[]  DifferentiatorOutMax=[]  FilterDiffOutCoefMin=[]  FilterDiffOutCoefMax=[]  ReciprocalOutMin=[]  ReciprocalOutMax=[]  SumDenOutMin=[]  SumDenOutMax=[]  SumNumOutMin=[]  SumNumOutMax=[]  DivideOutMin=[]  DivideOutMax=[]  UdiffTsProdOutMin=[]  UdiffTsProdOutMax=[]  NTsProdOutMin=[]  NTsProdOutMax=[]  UintegralTsProdOutMin=[]  UintegralTsProdOutMax=[]  UngainTsProdOutMin=[]  UngainTsProdOutMax=[]  IntegratorContinuousStateAttributes=''  IntegratorStateMustResolveToSignalObject=off  IntegratorRTWStateStorageClass=Auto  FilterContinuousStateAttributes=''  FilterStateMustResolveToSignalObject=off  FilterRTWStateStorageClass=Auto  ParallelPVariant=ExternalParameters  IdealPVariant=Disabled  IVariant=ExternalParameters  DVariant=ExternalParameters  IntegratorVariant=Discrete  SatVariant=Enabled  AWVariant=DiscClampingParallel  PCopyVariant=Disabled  TRVariant=Disabled  FdbkBlocksVariant=Forward  IdealPFdbkVariant=Disabled  SatFdbkVariant=Disabled  DerivativeFilterVariant=Differentiator  NVariant=Passthrough  NCopyVariant=Disabled_SignalSpec  FilterICVariant=InternalICsDifferentiator  IntegratorICVariant=InternalICs  ExternalResetVariant=Disabled  TRSumVariant=Passthrough  SumFdbkVariant=Disabled  SumVariant=Sum_PID  TsampFilterVariant=InternalTs  TsampNgainVariant=Passthrough  TsampIntegralVariant=Passthrough  ExternalSaturationOutDataTypeStr=Inherit: Same as second input
  Sum2 : Sum  Inputs=|+-
  pitch_cc : Outport
  wires:
  Sum2/1 -> Pitch angle controller/1  "pitch error"
  P_pitch_angle/1 -> Pitch angle controller/2
  I_pitch_angle/1 -> Pitch angle controller/3
  pitch_cmd_rad/1 -> Sum2/1  "pitch angle cmd"
  D_pitch_angle/1 -> Pitch angle controller/4
  Pitch angle controller/1 -> pitch_cc/1
  pitch_rad/1 -> Sum2/2

== system baseline_super/LAND CONTROLLER/Horizontal speed controller/Roll Controller ==
  roll_cmd_rad : Inport
  roll_rad : Inport  Port=2
  D_roll_angle : Constant  Value=Aircraft.Control.D_roll_angle  OutDataTypeStr=single
  I_roll_angle : Constant  Value=Aircraft.Control.I_roll_angle  OutDataTypeStr=single
  PID Controller1 : pid_lib/PID Controller  Controller=PID  Form=Parallel  TimeDomain=Discrete-time  UseExternalTs=off  SampleTime=framePeriod_s  IntegratorMethod=Forward Euler  FilterMethod=Forward Euler  ControllerParametersSource=external  P=0.335  I=0.005  D=0  UseFilter=off  N=100  TunerSelectOption=Transfer Function Based (PID Tuner App)  InitialConditionSource=internal  InitialConditionForIntegrator=0  InitialConditionForFilter=0  DifferentiatorICPrevScaledInput=0  ExternalReset=none  TrackingMode=off  Kt=1  LimitOutput=on  SatLimitsSource=internal  UpperSaturationLimit=inf  LowerSaturationLimit=-inf  LinearizeAsGain=off  AntiWindupMode=clamping  Kb=1  POutMin=[]  POutMax=[]  IOutMin=[]  IOutMax=[]  DOutMin=[]  DOutMax=[]  NOutMin=[]  NOutMax=[]  SumOutMin=[]  SumOutMax=[]  SaturationOutMin=[]  SaturationOutMax=[]  PParamMin=[]  PParamMax=[]  IParamMin=[]  IParamMax=[]  DParamMin=[]  DParamMax=[]  NParamMin=[]  NParamMax=[]  KbParamMin=[]  KbParamMax=[]  KtParamMin=[]  KtParamMax=[]  KbOutMin=[]  KbOutMax=[]  KtOutMin=[]  KtOutMax=[]  IntegratorOutMin=[]  IntegratorOutMax=[]  FilterOutMin=[]  FilterOutMax=[]  SumI1OutMin=[]  SumI1OutMax=[]  SumI2OutMin=[]  SumI2OutMax=[]  SumI3OutMin=[]  SumI3OutMax=[]  SumI4OutMin=[]  SumI4OutMax=[]  SumDOutMin=[]  SumDOutMax=[]  DifferentiatorOutMin=[]  DifferentiatorOutMax=[]  FilterDiffOutCoefMin=[]  FilterDiffOutCoefMax=[]  ReciprocalOutMin=[]  ReciprocalOutMax=[]  SumDenOutMin=[]  SumDenOutMax=[]  SumNumOutMin=[]  SumNumOutMax=[]  DivideOutMin=[]  DivideOutMax=[]  UdiffTsProdOutMin=[]  UdiffTsProdOutMax=[]  NTsProdOutMin=[]  NTsProdOutMax=[]  UintegralTsProdOutMin=[]  UintegralTsProdOutMax=[]  UngainTsProdOutMin=[]  UngainTsProdOutMax=[]  IntegratorContinuousStateAttributes=''  IntegratorStateMustResolveToSignalObject=off  IntegratorRTWStateStorageClass=Auto  FilterContinuousStateAttributes=''  FilterStateMustResolveToSignalObject=off  FilterRTWStateStorageClass=Auto  ParallelPVariant=ExternalParameters  IdealPVariant=Disabled  IVariant=ExternalParameters  DVariant=ExternalParameters  IntegratorVariant=Discrete  SatVariant=Enabled  AWVariant=DiscClampingParallel  PCopyVariant=Disabled  TRVariant=Disabled  FdbkBlocksVariant=Forward  IdealPFdbkVariant=Disabled  SatFdbkVariant=Disabled  DerivativeFilterVariant=Differentiator  NVariant=Passthrough  NCopyVariant=Disabled_SignalSpec  FilterICVariant=InternalICsDifferentiator  IntegratorICVariant=InternalICs  ExternalResetVariant=Disabled  TRSumVariant=Passthrough  SumFdbkVariant=Disabled  SumVariant=Sum_PID  TsampFilterVariant=InternalTs  TsampNgainVariant=Passthrough  TsampIntegralVariant=Passthrough  ExternalSaturationOutDataTypeStr=Inherit: Same as second input
  P_roll_angle : Constant  Value=Aircraft.Control.P_roll_angle  OutDataTypeStr=single
  Sum : Sum  Inputs=|+-
  roll_cc : Outport
  wires:
  PID Controller1/1 -> roll_cc/1  "Roll_cmd"
  roll_cmd_rad/1 -> Sum/1  "roll_angle_command"
  Sum/1 -> PID Controller1/1  "roll_angle_error"
  P_roll_angle/1 -> PID Controller1/2
  I_roll_angle/1 -> PID Controller1/3
  D_roll_angle/1 -> PID Controller1/4
  roll_rad/1 -> Sum/2
